simulink model "Test_rotgen_three_phase_s_function"  (Simulink 7.7)
settings: Solver=ode45  StartTime=0.0  StopTime=10.0  RelTol=1e-3
settings Model: Creator=s0237326  LastModifiedBy=s0237326

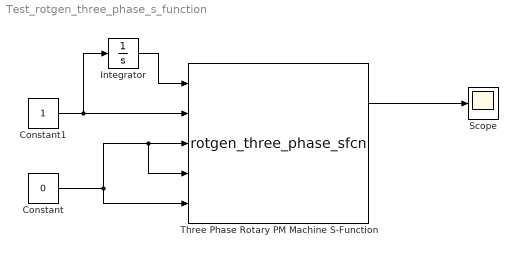
== system Test_rotgen_three_phase_s_function ==
  Constant : Constant  Value=0
  Constant1 : Constant
  Integrator : Integrator
  Scope : Scope
  Three Phase Rotary PM Machine S-Function : M-S-Function  FunctionName=rotgen_three_phase_sfcn
      mask Display:
      | port_label('input', 1, 'theta')
      | port_label('input', 2, 'omega')
      | port_label('input', 3, 'Phase A Current')
      | port_label('input', 4, 'Phase B Current')
      | port_label('input', 5, 'Phase C Current')
      | port_label('output', 1, 'Torque')
      | port_label('output', 2, 'Phase A EMF')
      | port_label('output', 3, 'Phase B EMF')
      | port_label('output', 4, 'Phase C EMF')
      | port_label('output', 5, 'Phase A Res')
      | port_label('output', 6, 'Phase B Res')
      | port_label('output', 7, 'Phase C Res')
  wires:
  Constant/1 -> Three Phase Rotary PM Machine S-Function/3, Three Phase Rotary PM Machine S-Function/4, Three Phase Rotary PM Machine S-Function/5
  Constant1/1 -> Three Phase Rotary PM Machine S-Function/2, Integrator/1
  Integrator/1 -> Three Phase Rotary PM Machine S-Function/1
  Three Phase Rotary PM Machine S-Function/2 -> Scope/1
